simulink model "EvPowertrainController2EM_r2_23a"  (R2023a)
settings: configuration reference "VehicleFixed10ms" (kept outside this file)
model workspace (MAT data in the model file):
  CtrlVcuAccelTrqScaleFctr = [0 0.5 0.8 1 1]
  CtrlVcuBattPnlty = 10000000
  CtrlVcuBattSOCBpts = [0 20 60 80 100]
  CtrlVcuCnstrntPnltyFctr = 10000000
  CtrlVcuEMPnlty = 100
  CtrlVcuEMTrqSplitGrid = 200
  CtrlVcuMaxAccelG = 1
  CtrlVcuMaxDecelG = -1.5
  CtrlVcuPwrDeltaPnlty = 10
  CtrlVcuRegenTrqScaleFctr = [1 0.8 0.5 0.3 0]
  CtrlVcuRoadMuEst = 0.8
  CtrlVcuSftyFctr = 0.9
  CtrlVcuTracPwrErrPnlty = 6
  CtrlVcuTrqVecBrkThresh = 0.01
  CtrlVcuTrqVecIGain = 0
  CtrlVcuTrqVecMinTrq = 25
  CtrlVcuTrqVecPGain = -2000
  CtrlVcuTrqVecSteerThresh = 0.349065850399
  CtrlVcuTrqVecVelThresh = 2.5
  N_P0 = 3
undefined symbols (not defined in the file): CtrlVcuEvChrgLmtBpt, CtrlVcuEvRegenBrkCutOff, CtrlVcuEvSocBpt, eff, EnvGrvty, PlntBrkActrBoreFrnt, PlntBrkFrntBias, PlntBrkKinFricCffFrnt, PlntBrkNumPadsFrnt, PlntBrkPadMeanRadiusFrnt, PlntBrkPrsFctr, PlntBrkRearBias, PlntDiffrntl2Eff, PlntDiffrntl2Ratio, PlntDiffrntlEff, PlntDiffrntlRatio, PlntEM1EffTbl, PlntEM1Spd, PlntEM1Trq, PlntEM1TrqEff, PlntEM2EffTbl, PlntEM2Spd, PlntEM2Trq, PlntEM2TrqEff, PlntEM3EffTbl, PlntEM3Spd, PlntEM3Trq, PlntEM3TrqEff, PlntEMWhlGearEffFL, PlntEMWhlGearEffRL, PlntEMWhlGearRatioFL, PlntEMWhlGearRatioRL, PlntTransEffSpdBpt, PlntTransEffTbl, PlntTransEffTempBpt, PlntTransEffTrqBpt, PlntTransGearNumVect, PlntTransGearRatioVect, PlntVehCGHgtAxl, PlntVehDstCGFrntAxl, PlntVehDstCGRearAxl, PlntVehMass, PlntWhlLdRadius, RegenEnd, RegenStrt
libraries: simulink x28, autolibutils x4, slpidlib x2
(part 6 of 6)

== system EvPowertrainController2EM_r2_23a/Energy Management/Powertrain Constraints /Wheel Torque Vector Logic/Regen/Wheel Torque Max Based on Power Limits/Power Management/Mech to Elec Power Estimate ==
  note: Pelec_req = Pmech_req*Eff^k,
      | k = -1 if Motoring >= 0,
      | k = 1 if Generating < 0
  note: Using an Efficiency Map, we can estimate the
      | Electric Power from the Mechanical  Torque Request.
  note: Check if Motoring
      | or Generating
  EMTrqCmd : Inport
  EMSpd : Inport  Port=2
  Abs : Abs  SaturateOnIntegerOverflow=off
  Abs1 : Abs  SaturateOnIntegerOverflow=off
  Constant1 : Constant  Value=-1  SampleTime=-1
  Constant2 : Constant  SampleTime=-1
  Eff Map : Lookup_n-D  BreakpointsForDimension1=PlntEM1Spd*30/pi  BreakpointsForDimension2=PlntEM1TrqEff  Table=PlntEM1EffTbl  ExtrapMethod=Clip  UseLastTableValue=on  InternalRulePriority=Speed  OutDataTypeStr=Inherit: Inherit from 'Table data'  RndMeth=Simplest
      settings: InputPortMap=u0,u1
  Gain1 : Gain  Gain=1/100
  Math Function : Math  Operator=pow  SignedPower=on  OutputSignalType=real
  Product : Product
  Product3 : Product
  Product4 : Product
  Switch2 : Switch  SaturateOnIntegerOverflow=off  InputSameDT=off
  rads_to_rpm : Gain  Gain=30/pi
  EMPwrElecReq : Outport  VectorParamsAs1DForOutWhenUnconnected=off
  Eff2k : Outport  Port=2  VectorParamsAs1DForOutWhenUnconnected=off
  wires:
  EMTrqCmd/1 -> Abs1/1, Product/2, Product3/2
  EMSpd/1 -> rads_to_rpm/1, Product/1, Product3/1
  Product/1 -> Switch2/2
  rads_to_rpm/1 -> Abs/1
  Abs1/1 -> Eff Map/2
  Product4/1 -> EMPwrElecReq/1
  Math Function/1 -> Product4/2, Eff2k/1
  Gain1/1 -> Math Function/1
  Abs/1 -> Eff Map/1
  Eff Map/1 -> Gain1/1
  Constant2/1 -> Switch2/3
  Constant1/1 -> Switch2/1
  Switch2/1 -> Math Function/2
  Product3/1 -> Product4/1

== system EvPowertrainController2EM_r2_23a/Energy Management/Powertrain Constraints /Wheel Torque Vector Logic/Regen/Wheel Torque Max Based on Power Limits/Power Management/Torque Limit ==
  EMTrq : Inport
  EMSpd : Inport  Port=2
  SOC : Inport  Port=3
  Compare To Constant : simulink/Logic and Bit Operations/Compare To Constant  relop=>  const=1  OutDataTypeStr=boolean
  Constant : Constant  Value=0  SampleTime=-1
  Gain : Gain  Gain=-1
  MaxEMTrqVsSpd : Lookup_n-D  NumberOfTableDimensions=1  BreakpointsForDimension1=PlntEM1Spd*30/pi  Table=PlntEM1Trq  ExtrapMethod=Clip  UseLastTableValue=on  InternalRulePriority=Speed  OutDataTypeStr=Inherit: Inherit from 'Table data'  RndMeth=Simplest
  Saturation Dynamic : simulink/Discontinuities/Saturation Dynamic  OutMin=[]  OutMax=[]  OutDataTypeStr=Inherit: Same as second input  OutDataType=fixdt(1, 16)  OutScaling=2^-10  DoSatur=off
  Switch : Switch  Criteria=u2 > Threshold  SaturateOnIntegerOverflow=off  InputSameDT=off
  rads_to_rpm : Gain  Gain=30/pi
  EMTrqCmd : Outport  VectorParamsAs1DForOutWhenUnconnected=off
  wires:
  Switch/1 -> Saturation Dynamic/1
  Constant/1 -> Switch/3
  Compare To Constant/1 -> Switch/2
  SOC/1 -> Compare To Constant/1
  Gain/1 -> Saturation Dynamic/3
  rads_to_rpm/1 -> MaxEMTrqVsSpd/1
  MaxEMTrqVsSpd/1 -> Switch/1, Gain/1
  EMSpd/1 -> rads_to_rpm/1
  Saturation Dynamic/1 -> EMTrqCmd/1
  EMTrq/1 -> Saturation Dynamic/2

== system EvPowertrainController2EM_r2_23a/Energy Management/Powertrain Constraints /Wheel Torque Vector Logic/Regen/Wheel Torque Max Based on Power Limits/WhlTrq2EMTrq/2EM or 3EM Dual Rear ==
  EMSpd : Inport
  WhlTrqCmd : Inport  Port=2
  Diff Eta : Subsystem
  Divide2 : Product  Inputs=/*
  Gain3 : Gain  Gain=1/PlntDiffrntlRatio
  Unit Delay : UnitDelay  SampleTime=-1  HasFrameUpgradeWarning=on
  EMTrq : Outport  VectorParamsAs1DForOutWhenUnconnected=off
  wires:
  Gain3/1 -> Divide2/2
  Divide2/1 -> Unit Delay/1, EMTrq/1
  EMSpd/1 -> Diff Eta/1(SpdIn)
  WhlTrqCmd/1 -> Gain3/1
  Diff Eta/1(eta) -> Divide2/1
  Unit Delay/1 -> Diff Eta/2(TrqIn)

== system EvPowertrainController2EM_r2_23a/Energy Management/Powertrain Constraints /Wheel Torque Vector Logic/Regen/Wheel Torque Max Based on Power Limits/WhlTrq2EMTrq/3EM Dual Front or 4EM ==
  EMSpd : Inport
  WhlTrqCmd : Inport  Port=2
  Divide2 : Product  Inputs=/*
  Dual EMs : Gain  Gain=1/2
  Gain3 : Gain  Gain=1/PlntEMWhlGearRatioFL
  Gear Eta : Subsystem
  Unit Delay : UnitDelay  SampleTime=-1  HasFrameUpgradeWarning=on
  EMTrq : Outport  VectorParamsAs1DForOutWhenUnconnected=off
  wires:
  Dual EMs/1 -> Gain3/1
  Gain3/1 -> Divide2/2
  Divide2/1 -> Unit Delay/1, EMTrq/1
  EMSpd/1 -> Gear Eta/1(SpdIn)
  WhlTrqCmd/1 -> Dual EMs/1
  Gear Eta/1(eta) -> Divide2/1
  Unit Delay/1 -> Gear Eta/2(TrqIn)

== system EvPowertrainController2EM_r2_23a/Energy Management/Powertrain Constraints /Wheel Torque Vector Logic/Traction/Wheel Torque Max Based on Power Limits/EMTrq2WhlTrq/2EM or 3EM Dual Front ==
  EMTrqCmd : Inport
  EMSpd : Inport  Port=2
  Diff Eta : Subsystem
  Divide2 : Product  Inputs=**
  Gain3 : Gain  Gain=PlntDiffrntl2Ratio
  WhlMotTrq : Outport  VectorParamsAs1DForOutWhenUnconnected=off
  wires:
  Diff Eta/1(eta) -> Divide2/1
  EMTrqCmd/1 -> Gain3/1, Diff Eta/2(TrqIn)
  EMSpd/1 -> Diff Eta/1(SpdIn)
  Divide2/1 -> WhlMotTrq/1
  Gain3/1 -> Divide2/2

== system EvPowertrainController2EM_r2_23a/Energy Management/Powertrain Constraints /Wheel Torque Vector Logic/Traction/Wheel Torque Max Based on Power Limits/EMTrq2WhlTrq/3EM Dual Rear or 4EM ==
  EMTrqCmd : Inport
  EMSpd : Inport  Port=2
  Divide2 : Product  Inputs=**
  Dual EMs : Gain  Gain=2
  Gain3 : Gain  Gain=PlntEMWhlGearRatioRL
  Gear Eta : Subsystem
  WhlMotTrq : Outport  VectorParamsAs1DForOutWhenUnconnected=off
  wires:
  Gear Eta/1(eta) -> Divide2/1
  EMTrqCmd/1 -> Dual EMs/1
  EMSpd/1 -> Gear Eta/1(SpdIn)
  Divide2/1 -> WhlMotTrq/1
  Gain3/1 -> Divide2/2
  Dual EMs/1 -> Gain3/1, Gear Eta/2(TrqIn)

== system EvPowertrainController2EM_r2_23a/Energy Management/Powertrain Constraints /Wheel Torque Vector Logic/Traction/Wheel Torque Max Based on Power Limits/Power Management/Check Within Limits ==
  up : Inport
  u : Inport  Port=2
  lo : Inport  Port=3
  Compare To Zero : simulink/Logic and Bit Operations/Compare To Zero  relop=>=  OutDataTypeStr=boolean
  Compare To Zero1 : simulink/Logic and Bit Operations/Compare To Zero  relop=<=  OutDataTypeStr=boolean
  Logical Operator : Logic  AllPortsSameDT=off  OutDataTypeStr=boolean
  Saturation Dynamic1 : simulink/Discontinuities/Saturation Dynamic  OutMin=[]  OutMax=[]  OutDataTypeStr=Inherit: Same as second input  OutDataType=fixdt(1, 16)  OutScaling=2^-10  DoSatur=off
  Subtract : Sum  Inputs=+-
  Subtract1 : Sum  Inputs=-+
  InLimit : Outport  VectorParamsAs1DForOutWhenUnconnected=off
  y : Outport  Port=2  VectorParamsAs1DForOutWhenUnconnected=off
  wires:
  Saturation Dynamic1/1 -> y/1
  lo/1 -> Subtract1/2, Saturation Dynamic1/3
  up/1 -> Subtract/1, Saturation Dynamic1/1
  u/1 -> Subtract1/1, Subtract/2, Saturation Dynamic1/2
  Subtract/1 -> Compare To Zero/1
  Subtract1/1 -> Compare To Zero1/1
  Compare To Zero/1 -> Logical Operator/1
  Compare To Zero1/1 -> Logical Operator/2
  Logical Operator/1 -> InLimit/1

== system EvPowertrainController2EM_r2_23a/Energy Management/Powertrain Constraints /Wheel Torque Vector Logic/Traction/Wheel Torque Max Based on Power Limits/Power Management/Mech to Elec Power Estimate ==
  note: Check if Motoring
      | or Generating
  note: Using an Efficiency Map, we can estimate the
      | Electric Power from the Mechanical  Torque Request.
  note: Pelec_req = Pmech_req*Eff^k,
      | k = -1 if Motoring >= 0,
      | k = 1 if Generating < 0
  EMTrqCmd : Inport
  EMSpd : Inport  Port=2
  Abs : Abs  SaturateOnIntegerOverflow=off
  Abs1 : Abs  SaturateOnIntegerOverflow=off
  Constant1 : Constant  Value=-1  SampleTime=-1
  Constant2 : Constant  SampleTime=-1
  Eff Map : Lookup_n-D  BreakpointsForDimension1=PlntEM2Spd*30/pi  BreakpointsForDimension2=PlntEM2TrqEff  Table=PlntEM2EffTbl  ExtrapMethod=Clip  UseLastTableValue=on  InternalRulePriority=Speed  OutDataTypeStr=Inherit: Inherit from 'Table data'  RndMeth=Simplest
      settings: InputPortMap=u0,u1
  Gain1 : Gain  Gain=1/100
  Math Function : Math  Operator=pow  SignedPower=on  OutputSignalType=real
  Product : Product
  Product3 : Product
  Product4 : Product
  Switch2 : Switch  SaturateOnIntegerOverflow=off  InputSameDT=off
  rads_to_rpm : Gain  Gain=30/pi
  EMPwrElecReq : Outport  VectorParamsAs1DForOutWhenUnconnected=off
  Eff2k : Outport  Port=2  VectorParamsAs1DForOutWhenUnconnected=off
  wires:
  Product3/1 -> Product4/1
  Switch2/1 -> Math Function/2
  Constant1/1 -> Switch2/1
  Constant2/1 -> Switch2/3
  Eff Map/1 -> Gain1/1
  Abs/1 -> Eff Map/1
  Gain1/1 -> Math Function/1
  Math Function/1 -> Eff2k/1, Product4/2
  Product4/1 -> EMPwrElecReq/1
  Abs1/1 -> Eff Map/2
  rads_to_rpm/1 -> Abs/1
  Product/1 -> Switch2/2
  EMSpd/1 -> Product3/1, Product/1, rads_to_rpm/1
  EMTrqCmd/1 -> Product3/2, Product/2, Abs1/1

== system EvPowertrainController2EM_r2_23a/Energy Management/Powertrain Constraints /Wheel Torque Vector Logic/Traction/Wheel Torque Max Based on Power Limits/Power Management/Torque Limit ==
  EMTrq : Inport
  EMSpd : Inport  Port=2
  SOC : Inport  Port=3
  Compare To Constant : simulink/Logic and Bit Operations/Compare To Constant  relop=>  const=1  OutDataTypeStr=boolean
  Constant : Constant  Value=0  SampleTime=-1
  Gain : Gain  Gain=-1
  MaxEMTrqVsSpd : Lookup_n-D  NumberOfTableDimensions=1  BreakpointsForDimension1=PlntEM2Spd*30/pi  Table=PlntEM2Trq  ExtrapMethod=Clip  UseLastTableValue=on  InternalRulePriority=Speed  OutDataTypeStr=Inherit: Inherit from 'Table data'  RndMeth=Simplest
  Saturation Dynamic : simulink/Discontinuities/Saturation Dynamic  OutMin=[]  OutMax=[]  OutDataTypeStr=Inherit: Same as second input  OutDataType=fixdt(1, 16)  OutScaling=2^-10  DoSatur=off
  Switch : Switch  Criteria=u2 > Threshold  SaturateOnIntegerOverflow=off  InputSameDT=off
  rads_to_rpm : Gain  Gain=30/pi
  EMTrqCmd : Outport  VectorParamsAs1DForOutWhenUnconnected=off
  wires:
  EMTrq/1 -> Saturation Dynamic/2
  Saturation Dynamic/1 -> EMTrqCmd/1
  EMSpd/1 -> rads_to_rpm/1
  MaxEMTrqVsSpd/1 -> Gain/1, Switch/1
  rads_to_rpm/1 -> MaxEMTrqVsSpd/1
  Gain/1 -> Saturation Dynamic/3
  SOC/1 -> Compare To Constant/1
  Compare To Constant/1 -> Switch/2
  Constant/1 -> Switch/3
  Switch/1 -> Saturation Dynamic/1

== system EvPowertrainController2EM_r2_23a/Energy Management/Powertrain Constraints /Wheel Torque Vector Logic/Traction/Wheel Torque Max Based on Power Limits/WhlTrq2EMTrq/2EM or 3EM Dual Front ==
  EMSpd : Inport
  WhlTrqCmd : Inport  Port=2
  Diff Eta : Subsystem
  Divide2 : Product  Inputs=/*
  Gain3 : Gain  Gain=1/PlntDiffrntl2Ratio
  Unit Delay : UnitDelay  SampleTime=-1  HasFrameUpgradeWarning=on
  EMTrq : Outport  VectorParamsAs1DForOutWhenUnconnected=off
  wires:
  Unit Delay/1 -> Diff Eta/2(TrqIn)
  Diff Eta/1(eta) -> Divide2/1
  WhlTrqCmd/1 -> Gain3/1
  EMSpd/1 -> Diff Eta/1(SpdIn)
  Divide2/1 -> EMTrq/1, Unit Delay/1
  Gain3/1 -> Divide2/2

== system EvPowertrainController2EM_r2_23a/Energy Management/Powertrain Constraints /Wheel Torque Vector Logic/Traction/Wheel Torque Max Based on Power Limits/WhlTrq2EMTrq/3EM Dual Rear or 4EM ==
  EMSpd : Inport
  WhlTrqCmd : Inport  Port=2
  Divide2 : Product  Inputs=/*
  Dual EMs : Gain  Gain=1/2
  Gain3 : Gain  Gain=1/PlntEMWhlGearRatioRL
  Gear Eta : Subsystem
  Unit Delay : UnitDelay  SampleTime=-1  HasFrameUpgradeWarning=on
  EMTrq : Outport  VectorParamsAs1DForOutWhenUnconnected=off
  wires:
  Dual EMs/1 -> Gain3/1
  Gain3/1 -> Divide2/2
  Divide2/1 -> Unit Delay/1, EMTrq/1
  EMSpd/1 -> Gear Eta/1(SpdIn)
  WhlTrqCmd/1 -> Dual EMs/1
  Gear Eta/1(eta) -> Divide2/1
  Unit Delay/1 -> Gear Eta/2(TrqIn)

== system EvPowertrainController2EM_r2_23a/Energy Management/Powertrain Constraints /Wheel Torque Vector Logic/Regen/Wheel Torque Max Based on Power Limits/EMTrq2WhlTrq/2EM or 3EM Dual Rear/Diff Eta ==
  note: Pwr >= 0, v = 1
      | Pwr < 0, v= -1
  SpdIn : Inport
  TrqIn : Inport  Port=2
  Constant : Constant  Value=PlntDiffrntl2Eff  SampleTime=-1
  Constant1 : Constant  SampleTime=-1
  Constant2 : Constant  Value=-1  SampleTime=-1
  Math Function1 : Math  Operator=pow  SignedPower=on  OutputSignalType=real
  Product1 : Product
  Switch2 : Switch  SaturateOnIntegerOverflow=off  InputSameDT=off
  eta : Outport  VectorParamsAs1DForOutWhenUnconnected=off
  wires:
  TrqIn/1 -> Product1/1
  Math Function1/1 -> eta/1
  Switch2/1 -> Math Function1/2
  Product1/1 -> Switch2/2
  Constant1/1 -> Switch2/1
  Constant2/1 -> Switch2/3
  Constant/1 -> Math Function1/1
  SpdIn/1 -> Product1/2

== system EvPowertrainController2EM_r2_23a/Energy Management/Powertrain Constraints /Wheel Torque Vector Logic/Regen/Wheel Torque Max Based on Power Limits/EMTrq2WhlTrq/3EM Dual Front or 4EM/Gear Eta ==
  note: Pwr >= 0, v = 1
      | Pwr < 0, v= -1
  SpdIn : Inport
  TrqIn : Inport  Port=2
  Constant : Constant  Value=PlntEMWhlGearEffFL
  Constant1 : Constant  SampleTime=-1
  Constant2 : Constant  Value=-1  SampleTime=-1
  Math Function1 : Math  Operator=pow  SignedPower=on  OutputSignalType=real
  Product1 : Product
  Switch2 : Switch  SaturateOnIntegerOverflow=off  InputSameDT=off
  eta : Outport  VectorParamsAs1DForOutWhenUnconnected=off
  wires:
  TrqIn/1 -> Product1/1
  Math Function1/1 -> eta/1
  Switch2/1 -> Math Function1/2
  Product1/1 -> Switch2/2
  Constant1/1 -> Switch2/1
  Constant2/1 -> Switch2/3
  Constant/1 -> Math Function1/1
  SpdIn/1 -> Product1/2

== system EvPowertrainController2EM_r2_23a/Energy Management/Powertrain Constraints /Wheel Torque Vector Logic/Regen/Wheel Torque Max Based on Power Limits/WhlTrq2EMTrq/2EM or 3EM Dual Rear/Diff Eta ==
  note: Pwr >= 0, v = 1
      | Pwr < 0, v= -1
  SpdIn : Inport
  TrqIn : Inport  Port=2
  Constant : Constant  Value=PlntDiffrntl2Eff  SampleTime=-1
  Constant1 : Constant  SampleTime=-1
  Constant2 : Constant  Value=-1  SampleTime=-1
  Math Function1 : Math  Operator=pow  SignedPower=on  OutputSignalType=real
  Product1 : Product
  Switch2 : Switch  SaturateOnIntegerOverflow=off  InputSameDT=off
  eta : Outport  VectorParamsAs1DForOutWhenUnconnected=off
  wires:
  TrqIn/1 -> Product1/1
  Math Function1/1 -> eta/1
  Switch2/1 -> Math Function1/2
  Product1/1 -> Switch2/2
  Constant1/1 -> Switch2/1
  Constant2/1 -> Switch2/3
  Constant/1 -> Math Function1/1
  SpdIn/1 -> Product1/2

== system EvPowertrainController2EM_r2_23a/Energy Management/Powertrain Constraints /Wheel Torque Vector Logic/Regen/Wheel Torque Max Based on Power Limits/WhlTrq2EMTrq/3EM Dual Front or 4EM/Gear Eta ==
  note: Pwr >= 0, v = 1
      | Pwr < 0, v= -1
  SpdIn : Inport
  TrqIn : Inport  Port=2
  Constant : Constant  Value=PlntEMWhlGearEffRL
  Constant1 : Constant  SampleTime=-1
  Constant2 : Constant  Value=-1  SampleTime=-1
  Math Function1 : Math  Operator=pow  SignedPower=on  OutputSignalType=real
  Product1 : Product
  Switch2 : Switch  SaturateOnIntegerOverflow=off  InputSameDT=off
  eta : Outport  VectorParamsAs1DForOutWhenUnconnected=off
  wires:
  TrqIn/1 -> Product1/1
  Math Function1/1 -> eta/1
  Switch2/1 -> Math Function1/2
  Product1/1 -> Switch2/2
  Constant1/1 -> Switch2/1
  Constant2/1 -> Switch2/3
  Constant/1 -> Math Function1/1
  SpdIn/1 -> Product1/2

== system EvPowertrainController2EM_r2_23a/Energy Management/Powertrain Constraints /Wheel Torque Vector Logic/Traction/Wheel Torque Max Based on Power Limits/EMTrq2WhlTrq/2EM or 3EM Dual Front/Diff Eta ==
  note: Pwr >= 0, v = 1
      | Pwr < 0, v= -1
  SpdIn : Inport
  TrqIn : Inport  Port=2
  Constant : Constant  Value=PlntDiffrntl2Eff  SampleTime=-1
  Constant1 : Constant  SampleTime=-1
  Constant2 : Constant  Value=-1  SampleTime=-1
  Math Function1 : Math  Operator=pow  SignedPower=on  OutputSignalType=real
  Product1 : Product
  Switch2 : Switch  SaturateOnIntegerOverflow=off  InputSameDT=off
  eta : Outport  VectorParamsAs1DForOutWhenUnconnected=off
  wires:
  SpdIn/1 -> Product1/2
  Constant/1 -> Math Function1/1
  Constant2/1 -> Switch2/3
  Constant1/1 -> Switch2/1
  Product1/1 -> Switch2/2
  Switch2/1 -> Math Function1/2
  Math Function1/1 -> eta/1
  TrqIn/1 -> Product1/1

== system EvPowertrainController2EM_r2_23a/Energy Management/Powertrain Constraints /Wheel Torque Vector Logic/Traction/Wheel Torque Max Based on Power Limits/EMTrq2WhlTrq/3EM Dual Rear or 4EM/Gear Eta ==
  note: Pwr >= 0, v = 1
      | Pwr < 0, v= -1
  SpdIn : Inport
  TrqIn : Inport  Port=2
  Constant : Constant  Value=PlntEMWhlGearEffRL
  Constant1 : Constant  SampleTime=-1
  Constant2 : Constant  Value=-1  SampleTime=-1
  Math Function1 : Math  Operator=pow  SignedPower=on  OutputSignalType=real
  Product1 : Product
  Switch2 : Switch  SaturateOnIntegerOverflow=off  InputSameDT=off
  eta : Outport  VectorParamsAs1DForOutWhenUnconnected=off
  wires:
  SpdIn/1 -> Product1/2
  Constant/1 -> Math Function1/1
  Constant2/1 -> Switch2/3
  Constant1/1 -> Switch2/1
  Product1/1 -> Switch2/2
  Switch2/1 -> Math Function1/2
  Math Function1/1 -> eta/1
  TrqIn/1 -> Product1/1

== system EvPowertrainController2EM_r2_23a/Energy Management/Powertrain Constraints /Wheel Torque Vector Logic/Traction/Wheel Torque Max Based on Power Limits/WhlTrq2EMTrq/2EM or 3EM Dual Front/Diff Eta ==
  note: Pwr >= 0, v = 1
      | Pwr < 0, v= -1
  SpdIn : Inport
  TrqIn : Inport  Port=2
  Constant : Constant  Value=PlntDiffrntl2Eff  SampleTime=-1
  Constant1 : Constant  SampleTime=-1
  Constant2 : Constant  Value=-1  SampleTime=-1
  Math Function1 : Math  Operator=pow  SignedPower=on  OutputSignalType=real
  Product1 : Product
  Switch2 : Switch  SaturateOnIntegerOverflow=off  InputSameDT=off
  eta : Outport  VectorParamsAs1DForOutWhenUnconnected=off
  wires:
  SpdIn/1 -> Product1/2
  Constant/1 -> Math Function1/1
  Constant2/1 -> Switch2/3
  Constant1/1 -> Switch2/1
  Product1/1 -> Switch2/2
  Switch2/1 -> Math Function1/2
  Math Function1/1 -> eta/1
  TrqIn/1 -> Product1/1

== system EvPowertrainController2EM_r2_23a/Energy Management/Powertrain Constraints /Wheel Torque Vector Logic/Traction/Wheel Torque Max Based on Power Limits/WhlTrq2EMTrq/3EM Dual Rear or 4EM/Gear Eta ==
  note: Pwr >= 0, v = 1
      | Pwr < 0, v= -1
  SpdIn : Inport
  TrqIn : Inport  Port=2
  Constant : Constant  Value=PlntEMWhlGearEffRL
  Constant1 : Constant  SampleTime=-1
  Constant2 : Constant  Value=-1  SampleTime=-1
  Math Function1 : Math  Operator=pow  SignedPower=on  OutputSignalType=real
  Product1 : Product
  Switch2 : Switch  SaturateOnIntegerOverflow=off  InputSameDT=off
  eta : Outport  VectorParamsAs1DForOutWhenUnconnected=off
  wires:
  TrqIn/1 -> Product1/1
  Math Function1/1 -> eta/1
  Switch2/1 -> Math Function1/2
  Product1/1 -> Switch2/2
  Constant1/1 -> Switch2/1
  Constant2/1 -> Switch2/3
  Constant/1 -> Math Function1/1
  SpdIn/1 -> Product1/2

== matlab function EvPowertrainController2EM_r2_23a/Energy Management/Hamiltonian computation and minimization/MATLAB Function ==
  data: minH output; idx output; H input; InfFlag input; allInf output
function [minH, idx, allInf] = fcn(H, InfFlag)

if all(InfFlag) 
    [minH, idx] = min(H);
    allInf = 1;
else
    [minH, idx] = min(H);
    allInf = 0;
end

== matlab function EvPowertrainController2EM_r2_23a/Torque Vectoring/4EM/Torque Vectoring Split Function Front ==
  data: MaxTrq input; TrqLeftOut output; TrqLeft input; TrqRght input; TrqRghtOut output; TrqVec input; Enbl input; BrkThresh input; MinTrq input
function [TrqLeftOut, TrqRghtOut] = fcn(MaxTrq, TrqLeft, TrqRght, TrqVec, Enbl, BrkThresh, MinTrq)
% Enbl:= flag to turn on TV, true if steering wheel is turned and non-zero vehicle speed
% BrkThresh:= flag to turn on TV, true if not braking
TrqLmt = min(MaxTrq-abs(TrqLeft),MaxTrq-abs(TrqRght));
DeltaTrq = min(MinTrq, min(TrqLmt,abs(TrqVec)))*sign(TrqVec)*Enbl;% limit difference in torque between tires to +/-MinTrq and to max/min motor torque
if BrkThresh > 0 % Not braking. Use Torque vectoring
    TrqLeftOut = (TrqLeft+DeltaTrq);
    TrqRghtOut = (TrqRght-DeltaTrq);
else % ignore TV
    TrqLeftOut = TrqLeft;
    TrqRghtOut = TrqRght;
end

== matlab function EvPowertrainController2EM_r2_23a/Torque Vectoring/3EM/Torque Vectoring Split Function ==
  data: MaxTrq input; TrqLeftOut output; TrqLeft input; TrqRght input; TrqRghtOut output; TrqVec input; Enbl input; BrkThresh input; MinTrq input
function [TrqLeftOut, TrqRghtOut] = fcn(MaxTrq, TrqLeft, TrqRght, TrqVec, Enbl, BrkThresh, MinTrq)
% Enbl:= flag to turn on TV, true if steering wheel is turned and non-zero vehicle speed
% BrkThresh:= flag to turn on TV, true if not braking
TrqLmt = min(MaxTrq-abs(TrqLeft),MaxTrq-abs(TrqRght));
DeltaTrq = min(MinTrq, min(TrqLmt,abs(TrqVec)))*sign(TrqVec)*Enbl;% limit difference in torque between tires to +/-MinTrq and to max/min motor torque
if BrkThresh > 0 % Not braking. Use Torque vectoring
    TrqLeftOut = (TrqLeft+DeltaTrq);
    TrqRghtOut = (TrqRght-DeltaTrq);
else % ignore TV
    TrqLeftOut = TrqLeft;
    TrqRghtOut = TrqRght;
end

== matlab function EvPowertrainController2EM_r2_23a/Torque Vectoring/4EM/Torque Vectoring Split Function Rear ==
  data: MaxTrq input; TrqLeftOut output; TrqLeft input; TrqRght input; TrqRghtOut output; TrqVec input; Enbl input; BrkThresh input; MinTrq input
function [TrqLeftOut, TrqRghtOut] = fcn(MaxTrq, TrqLeft, TrqRght, TrqVec, Enbl, BrkThresh, MinTrq)
% Enbl:= flag to turn on TV, true if steering wheel is turned and non-zero vehicle speed
% BrkThresh:= flag to turn on TV, true if not braking
TrqLmt = min(MaxTrq-abs(TrqLeft),MaxTrq-abs(TrqRght));
DeltaTrq = min(MinTrq, min(TrqLmt,abs(TrqVec)))*sign(TrqVec)*Enbl;% limit difference in torque between tires to +/-MinTrq and to max/min motor torque
if BrkThresh > 0 % Not braking. Use Torque vectoring
    TrqLeftOut = (TrqLeft+DeltaTrq);
    TrqRghtOut = (TrqRght-DeltaTrq);
else % ignore TV
    TrqLeftOut = TrqLeft;
    TrqRghtOut = TrqRght;
end
